simulink model "pitch_attitude_hold"  (R2017a)
settings: Solver=VariableStepAuto  StartTime=0.0  StopTime=10.0  RelTol=1e-3
values from neighbouring files (symbols this model uses):
  a_theta1 = -P.rho*Va^2*P.c*P.S_wing/(2*P.Jy)*P.C_m_q*P.c/(2*Va)    [computeRollGains.m]    (also in compute_gains.m)
  a_theta2 = -P.rho*Va^2*P.c*P.S_wing*P.C_m_alpha/(2*P.Jy)    [computeRollGains.m]    (also in compute_gains.m)
  a_theta3 = P.rho*Va^2*P.c*P.S_wing/(2*P.Jy)*P.C_m_delta_e    [computeRollGains.m]    (also in compute_gains.m)
  delta_e_max = 45*pi/180    (= 0.785398163397)    [computeRollGains.m]    (also in compute_gains.m = 0.523598775598)
  kd_theta = (2*zeta_theta*wn_theta - a_theta1)/a_theta3    [computeRollGains.m]
  kp_theta = delta_e_max/e_theta_max*sign(a_theta3)    [computeRollGains.m]
settings Model: Creator=pizzaslayer  LastModifiedBy=pizzaslayer

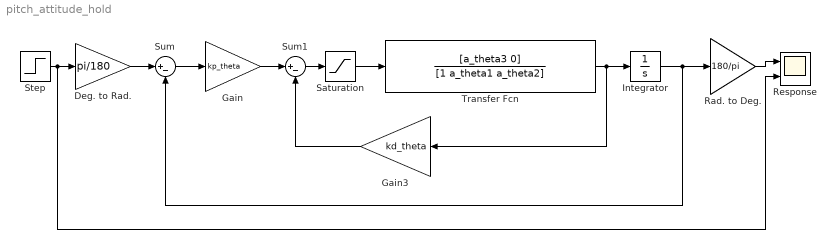
== system pitch_attitude_hold ==
  Deg. to Rad. : Gain  Gain=pi/180
  Gain : Gain  Gain=kp_theta
  Gain3 : Gain  Gain=kd_theta
  Integrator : Integrator
  Rad. to Deg. : Gain  Gain=180/pi
  Response : Scope  NumInputPorts=2
  Saturation : Saturate  UpperLimit=delta_e_max  LowerLimit=-delta_e_max
  Step : Step  Time=0  After=10  SampleTime=0
  Sum : Sum  Inputs=|+-
  Sum1 : Sum  Inputs=|+-
  Transfer Fcn : TransferFcn  Numerator=[a_theta3 0]  Denominator=[1 a_theta1 a_theta2]
  wires:
  Rad. to Deg./1 -> Response/1
  Step/1 -> Response/2, Deg. to Rad./1
  Deg. to Rad./1 -> Sum/1
  Sum/1 -> Gain/1
  Gain/1 -> Sum1/1
  Sum1/1 -> Saturation/1
  Saturation/1 -> Transfer Fcn/1
  Gain3/1 -> Sum1/2
  Transfer Fcn/1 -> Integrator/1, Gain3/1
  Integrator/1 -> Sum/2, Rad. to Deg./1
